simulink model "IPDISOsimNonlinearModel2015"  (R2013b)
settings: Solver=ode45  SolverMode=SingleTasking  StartTime=0.0  StopTime=20  FixedStep=0.001  RelTol=1e-3
settings Model: ExtModeTrigDuration=10000  Creator=eeuser  LastModifiedBy=eeyoyo
settings DataIOCC: LimitDataPoints=off  MaxDataPoints=100000  SaveFormat=StructureWithTime  SignalLoggingSaveFormat=ModelDataLogs  SignalLoggingName=sigsOut
settings OptimizationCC: BlockReduction=off  BooleanDataType=off  ExpressionDepthLimit=2147483647
settings DebuggingCC: SaveWithParameterizedLinksMsg=none  SignalResolutionControl=TryResolveAllWithWarning  SolverPrmCheckMsg=none  MultiTaskDSMMsg=warning  MultiTaskCondExecSysMsg=none  FcnCallInpInsideContextMsg=UseLocalSettings  StateNameClashWarn=warning
settings HardwareCC: ProdIntDivRoundTo=Zero  ProdEndianess=LittleEndian  ProdHWDeviceType=Generic->32-bit x86 compatible  TargetIntDivRoundTo=Zero  TargetEndianess=LittleEndian  TargetHWDeviceType=MATLAB Host  ProdEqTarget=off
settings RTWCC: SystemTargetFile=rtwin.tlc  TemplateMakefile=rtwin.tmf  ProcessScript=rtwin_make_rtw_hook  IncludeERTFirstTime=on  RTWCompilerOptimization=On
settings RTWinTargetCC: TargetLibSuffix=_rtwin.lib  TargetPreCompLibLocation=C:\Program Files\MATLAB\R2013b\toolbox\rtw\targets\rtwin\lib\win32  CodeReplacementLibrary=ANSI_C  RTWinDir=C:/PROGRA~1/MATLAB/R2013b/toolbox/rtw/targets/rtwin  TargetArch=win32

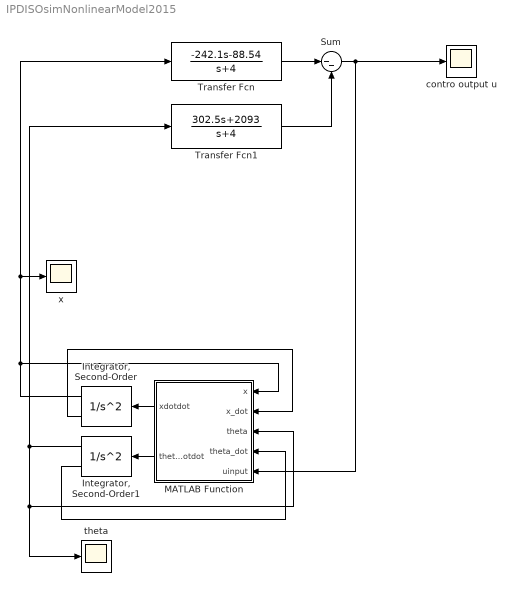
== system IPDISOsimNonlinearModel2015 ==
  "Integrator, Second-Order" : SecondOrderIntegrator  ICX=0.05  ICDXDT=5
  "Integrator, Second-Order1" : SecondOrderIntegrator  ICX=0.5  ICDXDT=1
  MATLAB Function : MATLAB Function  TreatAsAtomicUnit=on
  Sum : Sum  Inputs=|--  SaturateOnIntegerOverflow=on  InputSameDT=on  OutDataTypeStr=Inherit: Same as first input
  Transfer Fcn : TransferFcn  Numerator=[-242.1 -88.54]  Denominator=[1 4]
  Transfer Fcn1 : TransferFcn  Numerator=[302.5 2093]  Denominator=[1 4]
  contro output u : Scope
      settings: TickLabels=on  TimeRange=20  YMin=-1  YMax=1  SampleInput=on
  theta : Scope
      settings: TickLabels=on  TimeRange=20  YMax=15  SaveName=ScopeData4  SampleInput=on
  x : Scope
      settings: TickLabels=on  TimeRange=20  YMin=-2.75e+08  YMax=2.5e+07  SaveName=ScopeData2  SampleInput=on
  wires:
  "Integrator, Second-Order"/2 -> MATLAB Function/2(x_dot)
  "Integrator, Second-Order"/1 -> Transfer Fcn/1, x/1, MATLAB Function/1(x)
  MATLAB Function/1(xdotdot) -> "Integrator, Second-Order"/1
  MATLAB Function/2(thetadotdot) -> "Integrator, Second-Order1"/1
  "Integrator, Second-Order1"/2 -> MATLAB Function/4(theta_dot)
  Transfer Fcn/1 -> Sum/1
  Transfer Fcn1/1 -> Sum/2
  "Integrator, Second-Order1"/1 -> theta/1, MATLAB Function/3(theta), Transfer Fcn1/1
  Sum/1 -> contro output u/1, MATLAB Function/5(uinput)

== matlab function IPDISOsimNonlinearModel2015/MATLAB Function ==
  data: x input; xdotdot output; x_dot input; theta input; theta_dot input; uinput input; thetadotdot output
function [xdotdot,thetadotdot] = ipnonlinfcn(x,x_dot,theta,theta_dot,uinput)
%#codegen
%x=u(1)
%x_dot=u(2)
%theta=u(3)
%theta_dot=u(4)
%uinput=u(5)
Mp=0.2107;
Mc=0.51;
g=9.8;
L=0.61;
Kg=14/1;
Kb=0.00767;
Ra=3;
R=0.008;
A=[Mc+Mp,-1/2*Mp*L*cos(theta);-cos(theta), 2/3*L];
y=inv(A)*[Kb*Kg*uinput/(Ra*R)-Kb^2*Kg^2*x_dot/(Ra*R^2)-1/2*Mp*L*theta_dot^2*sin(theta);g*sin(theta)];
xdotdot=y(1);
thetadotdot=y(2);

;
